simulink model "linear_approx"  (R2020b)
settings: Solver=VariableStepAuto  StartTime=0.0  StopTime=10.0  RelTol=1e-3
values from neighbouring files (symbols this model uses):
  D0 = 0    [simulation.m]
  dE0 = E0    (= 0.145)    [simulation.m]
  dI0 = I0    (= 0.05)    [simulation.m]
  dJ0 = J0    (= 0.005)    [simulation.m]
  dR0 = R0    (= 0)    [simulation.m]
  dS0 = S0    (= 0.8)    [simulation.m]
  Se = 0.1    [simulation.m]
settings Model: Creator=leumas  LastModifiedBy=leumas

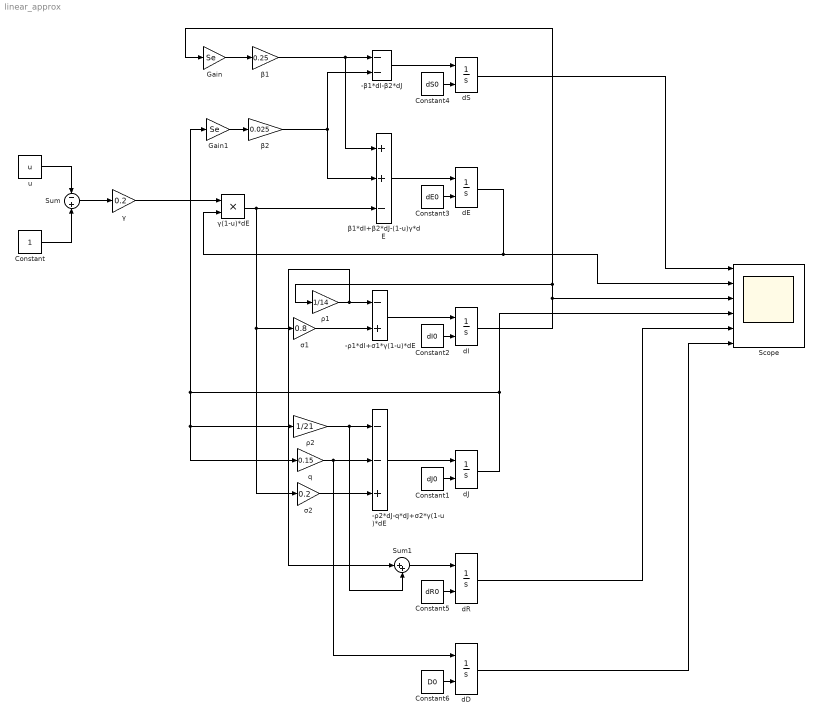
== system linear_approx ==
  -β1*dI-β2*dJ : Sum  Inputs=--
  -ρ1*dI+σ1*γ(1-u)*dE : Sum  Inputs=-+
  -ρ2*dJ-q*dJ+σ2*γ(1-u)*dE : Sum  Inputs=--+
  Constant : Constant
  Constant1 : Constant  Value=dJ0
  Constant2 : Constant  Value=dI0
  Constant3 : Constant  Value=dE0
  Constant4 : Constant  Value=dS0
  Constant5 : Constant  Value=dR0
  Constant6 : Constant  Value=D0
  Gain : Gain  Gain=Se
  Gain1 : Gain  Gain=Se
  Scope : Scope  NumInputPorts=6
  Sum : Sum  Inputs=-+
  Sum1 : Sum  Inputs=|++
  dD : Integrator  InitialConditionSource=external
  dE : Integrator  InitialConditionSource=external
  dI : Integrator  InitialConditionSource=external
  dJ : Integrator  InitialConditionSource=external
  dR : Integrator  InitialConditionSource=external
  dS : Integrator  InitialConditionSource=external
  "q  " : Gain  Gain=0.15
  u : Constant  Value=u
  "β1 " : Gain  Gain=0.25
  β1*dI+β2*dJ-(1-u)γ*dE : Sum  Inputs=++-
  "β2  " : Gain  Gain=0.025
  "γ   " : Gain  Gain=0.2
  γ(1-u)*dE : Product
  "ρ1  " : Gain  Gain=1/14
  "ρ2  " : Gain  Gain=1/21
  "σ1 " : Gain  Gain=0.8
  "σ2 " : Gain  Gain=0.2
  wires:
  dD/1 -> Scope/6
  Constant/1 -> Sum/2
  "ρ1  "/1 -> Sum1/1, -ρ1*dI+σ1*γ(1-u)*dE/1
  Gain/1 -> "β1 "/1
  Gain1/1 -> "β2  "/1
  dI/1 -> Scope/3, Gain/1, "ρ1  "/1
  -ρ2*dJ-q*dJ+σ2*γ(1-u)*dE/1 -> dJ/1
  "β2  "/1 -> -β1*dI-β2*dJ/2, β1*dI+β2*dJ-(1-u)γ*dE/2
  Sum1/1 -> dR/1
  Constant6/1 -> dD/2
  Constant5/1 -> dR/2
  Constant3/1 -> dE/2
  dE/1 -> Scope/2, γ(1-u)*dE/2
  "σ1 "/1 -> -ρ1*dI+σ1*γ(1-u)*dE/2
  γ(1-u)*dE/1 -> β1*dI+β2*dJ-(1-u)γ*dE/3, "σ2 "/1, "σ1 "/1
  -ρ1*dI+σ1*γ(1-u)*dE/1 -> dI/1
  Constant4/1 -> dS/2
  dR/1 -> Scope/5
  "γ   "/1 -> γ(1-u)*dE/1
  "ρ2  "/1 -> -ρ2*dJ-q*dJ+σ2*γ(1-u)*dE/1, Sum1/2
  "β1 "/1 -> -β1*dI-β2*dJ/1, β1*dI+β2*dJ-(1-u)γ*dE/1
  dJ/1 -> Scope/4, Gain1/1, "q  "/1, "ρ2  "/1
  Constant2/1 -> dI/2
  "σ2 "/1 -> -ρ2*dJ-q*dJ+σ2*γ(1-u)*dE/3
  -β1*dI-β2*dJ/1 -> dS/1
  u/1 -> Sum/1
  Constant1/1 -> dJ/2
  "q  "/1 -> -ρ2*dJ-q*dJ+σ2*γ(1-u)*dE/2, dD/1
  dS/1 -> Scope/1
  Sum/1 -> "γ   "/1
  β1*dI+β2*dJ-(1-u)γ*dE/1 -> dE/1
